simulink model "s_func_drone_vid2_fastest"
settings: Solver=FixedStepDiscrete  StartTime=0.0  StopTime=inf  FixedStep=0.05  RelTol=1e-3
libraries: etargetslib x12, dspnetwork x9, xpcseriallib x7, dspmtrx3 x4, visionsinks x1
settings Model: Creator=Ballistyx  LastModifiedBy=JLEE
settings DataIOCC: LimitDataPoints=on  SaveFormat=Array  SignalLoggingSaveFormat=ModelDataLogs  ReturnWorkspaceOutputs=off
settings OptimizationCC: ExpressionDepthLimit=2147483647  LifeSpan=inf  SimCompilerOptimization=Off
settings DebuggingCC: UnderspecifiedInitializationDetection=Classic  MergeDetectMultiDrivingBlocksExec=none  SolverPrmCheckMsg=warning  MultiTaskDSMMsg=warning  MultiTaskCondExecSysMsg=none  FcnCallInpInsideContextMsg=Enable All  FrameProcessingCompatibilityMsg=warning  StateNameClashWarn=warning  StrictBusMsg=None  SFUnexpectedBacktrackingDiag=warning  SFNoUnconditionalDefaultTransitionDiag=warning
settings HardwareCC: ProdBitPerPointer=32  ProdLargestAtomicFloat=None  ProdIntDivRoundTo=Undefined  ProdEndianess=Unspecified  ProdWordSize=32  ProdHWDeviceType=32-bit Generic
settings ModelReferenceCC: PropagateSignalLabelsOutOfModel=off
settings SFSimCC: SimUseLocalCustomCode=off
settings RTWCC: RTWUseLocalCustomCode=off  IncludeERTFirstTime=on  RTWCompilerOptimization=Off
settings CodeAppCC: CustomSymbolStrType=$N$R$M
settings GRTTargetCC: CodeReplacementLibrary=ANSI_C  GeneratePreprocessorConditionals=Disable all  CPPClassGenCompliant=off

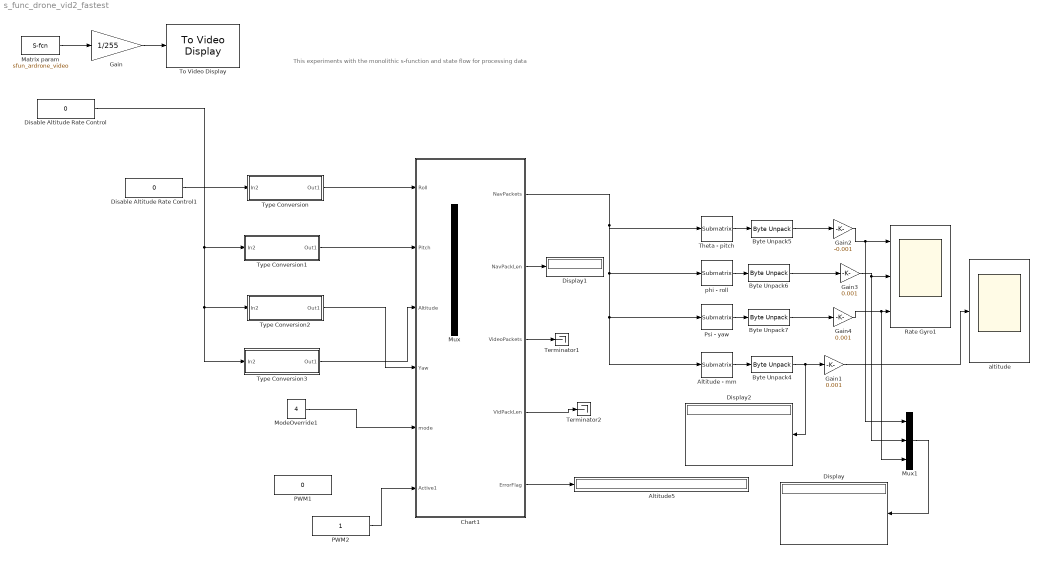
== system s_func_drone_vid2_fastest ==
  note: This experiments with the monolithic s-function and state flow for processing data
  Altitude - mm : dspmtrx3/Submatrix  RowSpan=Range of rows  RowStartMode=Index  RowStartIndex=41  RowEndMode=Index  RowEndIndex=44  ColSpan=All columns  ColStartMode=Index  ColStartIndex=4  ColEndMode=Index  ColEndIndex=4
  Altitude5 : Display
  Byte Unpack4 : etargetslib/Byte Unpack  dimensions={[1]}  datatypes={'uint32'}  byteAlign=1
  Byte Unpack5 : etargetslib/Byte Unpack  dimensions={[1]}  datatypes={'single'}  byteAlign=1
  Byte Unpack6 : etargetslib/Byte Unpack  dimensions={[1]}  datatypes={'single'}  byteAlign=1
  Byte Unpack7 : etargetslib/Byte Unpack  dimensions={[1]}  datatypes={'single'}  byteAlign=1
  Chart1 : Stateflow chart  TreatAsAtomicUnit=on
  Disable Altitude Rate Control : Constant  Value=0
  Disable Altitude Rate Control1 : Constant  Value=0
  Display : Display
  Display1 : Display
  Display2 : Display
  Gain : Gain  Gain=1/255
  Gain1 : Gain  Gain=0.001
  Gain2 : Gain  Gain=-0.001
  Gain3 : Gain  Gain=0.001
  Gain4 : Gain  Gain=0.001
  Matrix param : S-Function  FunctionName=sfun_ardrone_video  Parameters=Operand  EnableBusSupport=off  mask(Matrix add){Operand=4}
      mask prompts: Operand "Operand 1:"
      settings: AttributesFormatString=Param = %<Operand>
      mask Display: disp('Matrix\n Add ')
  ModeOverride1 : Constant  Value=4
  Mux : Mux
  Mux1 : Mux  Inputs=3
  PWM1 : Constant  Value=0
  PWM2 : Constant
  Psi - yaw : dspmtrx3/Submatrix  RowSpan=Range of rows  RowStartMode=Index  RowStartIndex=37  RowEndMode=Index  RowEndIndex=40  ColSpan=All columns  ColStartMode=Index  ColStartIndex=4  ColEndMode=Index  ColEndIndex=4
  Rate Gyro1 : Scope  NumInputPorts=3
      settings: YMin=0.295~2.935~32.9  YMax=0.365~3~34.4  SaveName=NavData_Simulink1
  Terminator1 : Terminator
  Terminator2 : Terminator
  Theta - pitch : dspmtrx3/Submatrix  RowSpan=Range of rows  RowStartMode=Index  RowStartIndex=29  RowEndMode=Index  RowEndIndex=32  ColSpan=All columns  ColStartMode=Index  ColStartIndex=4  ColEndMode=Index  ColEndIndex=4
  To Video Display : visionsinks/To Video Display  inputType=Obsolete  imagePorts=One multidimensional signal  OutputDevice=On-screen video monitor  fullScreen=off  videoWindowX=223  videoWindowY=316  saveWindowSize=off  videoWindowWidth=320  videoWindowHeight=240  dataOrg=Column-major  openAtMdlStart=on  isWindowOpen=on  inputColorFormat=RGB
  Type Conversion : Subsystem
  Type Conversion1 : Subsystem
  Type Conversion2 : Subsystem
  Type Conversion3 : Subsystem
  altitude : Scope
      settings: YMin=0.242  YMax=0.242  SaveName=NavData_Simulink
  phi - roll : dspmtrx3/Submatrix  RowSpan=Range of rows  RowStartMode=Index  RowStartIndex=33  RowEndMode=Index  RowEndIndex=36  ColSpan=All columns  ColStartMode=Index  ColStartIndex=4  ColEndMode=Index  ColEndIndex=4
  wires:
  Matrix param/1 -> Gain/1
  Gain/1 -> To Video Display/1
  Altitude - mm/1 -> Byte Unpack4/1
  Theta - pitch/1 -> Byte Unpack5/1
  phi - roll/1 -> Byte Unpack6/1
  Psi - yaw/1 -> Byte Unpack7/1
  Byte Unpack5/1 -> Gain2/1
  Byte Unpack6/1 -> Gain3/1
  Byte Unpack7/1 -> Gain4/1
  Byte Unpack4/1 -> Gain1/1, Display2/1
  Gain1/1 -> altitude/1
  Gain2/1 -> Rate Gyro1/1, Mux1/1
  Gain3/1 -> Rate Gyro1/2, Mux1/2
  Gain4/1 -> Rate Gyro1/3, Mux1/3
  PWM2/1 -> Chart1/6(Active1)
  Chart1/4(VidPackLen) -> Terminator2/1
  Chart1/5(ErrorFlag) -> Altitude5/1
  Type Conversion3/1(Out1) -> Chart1/3(Altitude)
  Type Conversion2/1(Out1) -> Chart1/4(Yaw)
  Type Conversion1/1(Out1) -> Chart1/2(Pitch)
  Type Conversion/1(Out1) -> Chart1/1(Roll)
  Disable Altitude Rate Control1/1 -> Type Conversion/1(In2)
  Disable Altitude Rate Control/1 -> Type Conversion1/1(In2), Type Conversion3/1(In2), Type Conversion2/1(In2)
  ? -> ?
  ModeOverride1/1 -> Chart1/5(mode)
  Chart1/2(NavPackLen) -> Display1/1
  Chart1/3(VideoPackets) -> Terminator1/1
  Chart1/1(NavPackets) -> Theta - pitch/1, phi - roll/1, Psi - yaw/1, Altitude - mm/1
  Mux1/1 -> Display/1

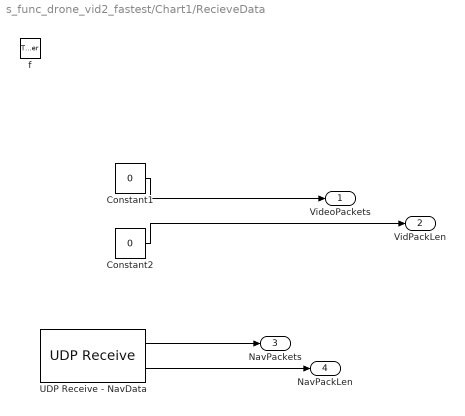
== system s_func_drone_vid2_fastest/Chart1/RecieveData ==
  f : TriggerPort  TriggerType=function-call
      settings: CopyFcn=Stateflow.SLINSF.SimulinkMan.removeBlockPreDeleteFcn  PreDeleteFcn=Stateflow.SLINSF.SimulinkMan.unsafePredeleteFcn
  Constant1 : Constant  Value=0
  Constant2 : Constant  Value=0
  UDP Receive - NavData : dspnetwork/UDP Receive  Priority=11  localURL='0.0.0.0'  localPort=5554  remoteURL='192.168.1.1'  remotePort=-1  recvBufferSize=500  dims=500  signalDatatype=uint8  isVarSize=off  showBlockingTime=off  blockingTime=0  sampletime=-1
  VideoPackets : Outport
  VidPackLen : Outport  Port=2
  NavPackets : Outport  Port=3
  NavPackLen : Outport  Port=4
  wires:
  Constant1/1 -> VideoPackets/1
  Constant2/1 -> VidPackLen/1
  UDP Receive - NavData/1 -> NavPackets/1
  UDP Receive - NavData/2 -> NavPackLen/1

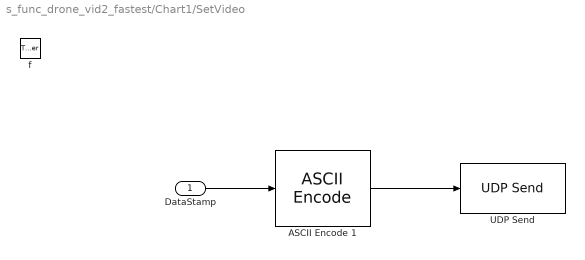
== system s_func_drone_vid2_fastest/Chart1/SetVideo ==
  DataStamp : Inport
  f : TriggerPort  TriggerType=function-call
      settings: CopyFcn=Stateflow.SLINSF.SimulinkMan.removeBlockPreDeleteFcn  PreDeleteFcn=Stateflow.SLINSF.SimulinkMan.unsafePredeleteFcn
  ASCII Encode 1 : xpcseriallib/ASCII Encode   format="AT*CONFIG=%d,\\\"video:video_channel\\\",\\\"0\\\"\\r"  nvars=1  maxlength=44  vartypes={ 'uint32' }
  UDP Send : dspnetwork/UDP Send  remoteURL='192.168.1.1'  remotePort=5556  localURL='0.0.0.0'  localPortSource=Specify via dialog  localPort=5556  sampletime=-1  separateLengthPort=0
  wires:
  DataStamp/1 -> ASCII Encode 1/1
  ASCII Encode 1/1 -> UDP Send/1

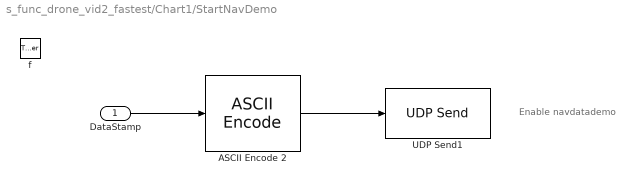
== system s_func_drone_vid2_fastest/Chart1/StartNavDemo ==
  note: Enable navdatademo
  DataStamp : Inport
  f : TriggerPort  TriggerType=function-call
      settings: CopyFcn=Stateflow.SLINSF.SimulinkMan.removeBlockPreDeleteFcn  PreDeleteFcn=Stateflow.SLINSF.SimulinkMan.unsafePredeleteFcn
  ASCII Encode 2 : xpcseriallib/ASCII Encode   format="AT*CONFIG=%d,\\\"general:navdata_demo\\\",\\\"TRUE\\\"\\r"  nvars=1  maxlength=43  vartypes={ 'uint32' }
  UDP Send1 : dspnetwork/UDP Send  remoteURL='192.168.1.1'  remotePort=5556  localURL='0.0.0.0'  localPortSource=Specify via dialog  localPort=5556  sampletime=-1  separateLengthPort=0
  wires:
  DataStamp/1 -> ASCII Encode 2/1
  ASCII Encode 2/1 -> UDP Send1/1

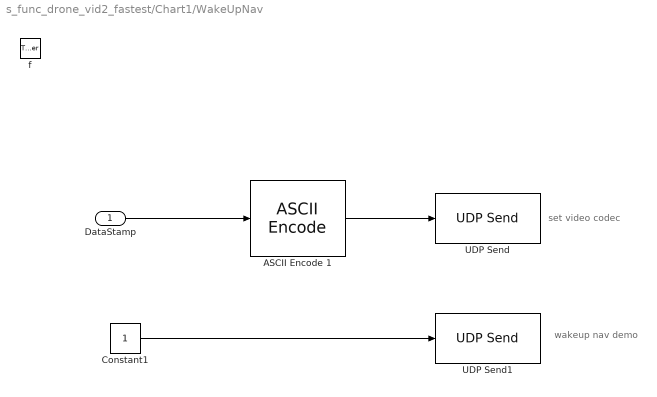
== system s_func_drone_vid2_fastest/Chart1/WakeUpNav ==
  note: set video codec
  note: wakeup nav demo
  DataStamp : Inport
  f : TriggerPort  TriggerType=function-call
      settings: CopyFcn=Stateflow.SLINSF.SimulinkMan.removeBlockPreDeleteFcn  PreDeleteFcn=Stateflow.SLINSF.SimulinkMan.unsafePredeleteFcn
  ASCII Encode 1 : xpcseriallib/ASCII Encode   format="AT*CONFIG=%d,\\\"video:video_codec\\\",\\\"32\\\"\\r"  nvars=1  maxlength=44  vartypes={ 'uint32' }
  Constant1 : Constant  OutDataTypeStr=uint8  SampleTime=-1
  UDP Send : dspnetwork/UDP Send  remoteURL='192.168.1.1'  remotePort=5556  localURL='0.0.0.0'  localPortSource=Specify via dialog  localPort=5556  sampletime=-1  separateLengthPort=0
  UDP Send1 : dspnetwork/UDP Send  remoteURL='192.168.1.1'  remotePort=5554  localURL='0.0.0.0'  localPortSource=Specify via dialog  localPort=5554  sampletime=-1  separateLengthPort=0
  wires:
  DataStamp/1 -> ASCII Encode 1/1
  Constant1/1 -> UDP Send1/1
  ASCII Encode 1/1 -> UDP Send/1

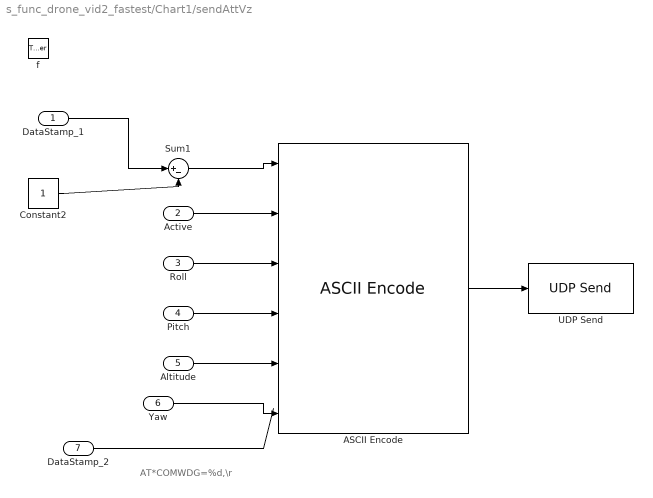
== system s_func_drone_vid2_fastest/Chart1/sendAttVz ==
  note: AT*COMWDG=%d,\r
  DataStamp_1 : Inport
  Active : Inport  Port=2
  Roll : Inport  Port=3
  Pitch : Inport  Port=4
  Altitude : Inport  Port=5
  Yaw : Inport  Port=6
  DataStamp_2 : Inport  Port=7
  f : TriggerPort  TriggerType=function-call
      settings: CopyFcn=Stateflow.SLINSF.SimulinkMan.removeBlockPreDeleteFcn  PreDeleteFcn=Stateflow.SLINSF.SimulinkMan.unsafePredeleteFcn
  "ASCII Encode " : xpcseriallib/ASCII Encode   format=AT*PCMD=%d,%d,%d,%d,%d,%d\r  nvars=6  maxlength=128  vartypes={ 'double' }
  Constant2 : Constant
  Sum1 : Sum  Inputs=|+-
  UDP Send : dspnetwork/UDP Send  remoteURL='192.168.1.1'  remotePort=5556  localURL='0.0.0.0'  localPortSource=Specify via dialog  localPort=5556  sampletime=-1  separateLengthPort=0
  wires:
  Active/1 -> "ASCII Encode "/2
  Roll/1 -> "ASCII Encode "/3
  Pitch/1 -> "ASCII Encode "/4
  Altitude/1 -> "ASCII Encode "/5
  Yaw/1 -> "ASCII Encode "/6
  DataStamp_2/1 -> ?
  DataStamp_1/1 -> Sum1/1
  Sum1/1 -> "ASCII Encode "/1
  Constant2/1 -> Sum1/2
  "ASCII Encode "/1 -> UDP Send/1

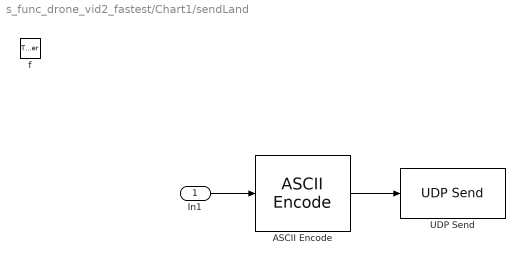
== system s_func_drone_vid2_fastest/Chart1/sendLand ==
  In1 : Inport
  f : TriggerPort  TriggerType=function-call
      settings: CopyFcn=Stateflow.SLINSF.SimulinkMan.removeBlockPreDeleteFcn  PreDeleteFcn=Stateflow.SLINSF.SimulinkMan.unsafePredeleteFcn
  "ASCII Encode " : xpcseriallib/ASCII Encode   format=AT*REF=%d,290717696\r  nvars=1  maxlength=128  vartypes={ 'double' }
  UDP Send : dspnetwork/UDP Send  remoteURL='192.168.1.1'  remotePort=5556  localURL='0.0.0.0'  localPortSource=Specify via dialog  localPort=5556  sampletime=-1  separateLengthPort=0
  wires:
  "ASCII Encode "/1 -> UDP Send/1
  In1/1 -> "ASCII Encode "/1

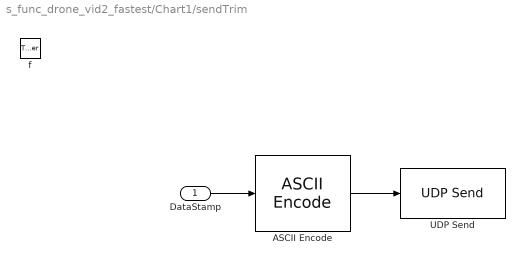
== system s_func_drone_vid2_fastest/Chart1/sendTrim ==
  DataStamp : Inport
  f : TriggerPort  TriggerType=function-call
      settings: CopyFcn=Stateflow.SLINSF.SimulinkMan.removeBlockPreDeleteFcn  PreDeleteFcn=Stateflow.SLINSF.SimulinkMan.unsafePredeleteFcn
  "ASCII Encode " : xpcseriallib/ASCII Encode   format=AT*FTRIM=%d,\r  nvars=1  maxlength=128  vartypes={ 'double' }
  UDP Send : dspnetwork/UDP Send  remoteURL='192.168.1.1'  remotePort=5556  localURL='0.0.0.0'  localPortSource=Specify via dialog  localPort=5556  sampletime=-1  separateLengthPort=0
  wires:
  "ASCII Encode "/1 -> UDP Send/1
  DataStamp/1 -> "ASCII Encode "/1

== system s_func_drone_vid2_fastest/Chart1/startHover ==
  note: disable hover for now
  DataStamp : Inport
  f : TriggerPort  TriggerType=function-call
      settings: CopyFcn=Stateflow.SLINSF.SimulinkMan.removeBlockPreDeleteFcn  PreDeleteFcn=Stateflow.SLINSF.SimulinkMan.unsafePredeleteFcn
  "ASCII Encode " : xpcseriallib/ASCII Encode   format=AT*REF=%d,290718208\r  nvars=1  maxlength=128  vartypes={ 'double' }
  UDP Send : dspnetwork/UDP Send  remoteURL='192.168.1.1'  remotePort=5556  localURL='0.0.0.0'  localPortSource=Specify via dialog  localPort=5556  sampletime=-1  separateLengthPort=0
  wires:
  DataStamp/1 -> "ASCII Encode "/1

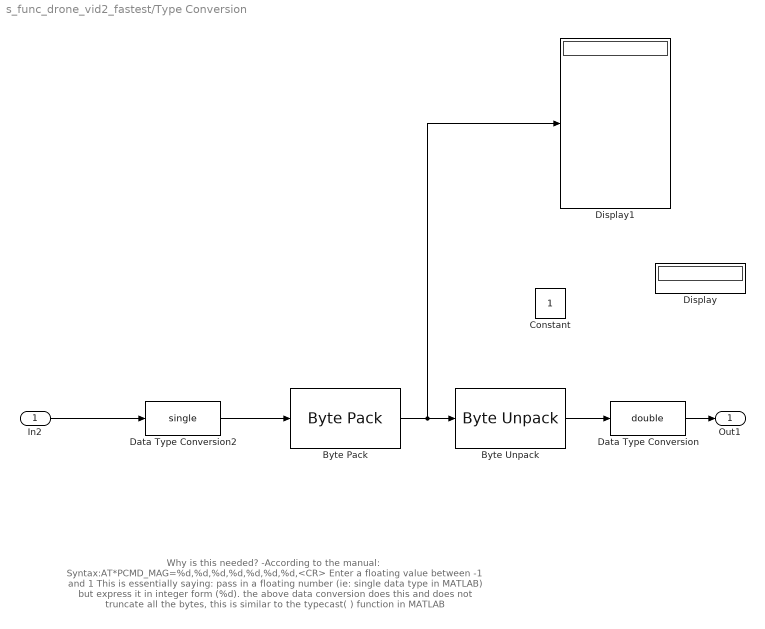
== system s_func_drone_vid2_fastest/Type Conversion ==
  note: Why is this needed?
      | -According to the manual:
      |
      | Syntax:AT*PCMD_MAG=%d,%d,%d,%d,%d,%d,%d,<CR>
      | Enter a floating value between -1 and 1
      |
      | This is essentially saying: pass in a floating number (ie: single data type in MATLAB) but express it in integer form (%d).
      | the above data conversion does this and does not truncate all the bytes, this is similar to the typecast( ) function in MATLAB
  In2 : Inport
  Byte Pack : etargetslib/Byte Pack  datatypes={'single'}  byteAlign=1
  Byte Unpack : etargetslib/Byte Unpack  dimensions={[1]}  datatypes={'int32'}  byteAlign=1
  Constant : Constant
  Data Type Conversion : DataTypeConversion  OutDataTypeStr=double
  Data Type Conversion2 : DataTypeConversion  OutDataTypeStr=single
  Display : Display
  Display1 : Display
  Out1 : Outport
  wires:
  In2/1 -> Data Type Conversion2/1
  Data Type Conversion2/1 -> Byte Pack/1
  Data Type Conversion/1 -> Out1/1
  Byte Pack/1 -> Byte Unpack/1, Display1/1
  Byte Unpack/1 -> Data Type Conversion/1
  ? -> Display/1

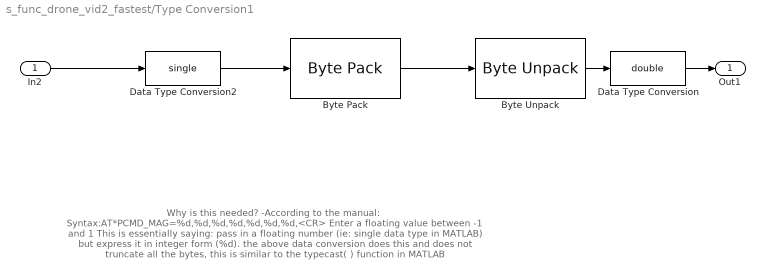
== system s_func_drone_vid2_fastest/Type Conversion1 ==
  note: Why is this needed?
      | -According to the manual:
      |
      | Syntax:AT*PCMD_MAG=%d,%d,%d,%d,%d,%d,%d,<CR>
      | Enter a floating value between -1 and 1
      |
      | This is essentially saying: pass in a floating number (ie: single data type in MATLAB) but express it in integer form (%d).
      | the above data conversion does this and does not truncate all the bytes, this is similar to the typecast( ) function in MATLAB
  In2 : Inport
  Byte Pack : etargetslib/Byte Pack  datatypes={'single'}  byteAlign=1
  Byte Unpack : etargetslib/Byte Unpack  dimensions={[1]}  datatypes={'int32'}  byteAlign=1
  Data Type Conversion : DataTypeConversion  OutDataTypeStr=double
  Data Type Conversion2 : DataTypeConversion  OutDataTypeStr=single
  Out1 : Outport
  wires:
  Byte Pack/1 -> Byte Unpack/1
  Byte Unpack/1 -> Data Type Conversion/1
  In2/1 -> Data Type Conversion2/1
  Data Type Conversion2/1 -> Byte Pack/1
  Data Type Conversion/1 -> Out1/1

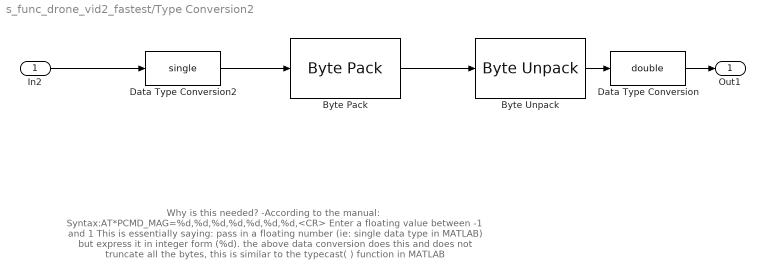
== system s_func_drone_vid2_fastest/Type Conversion2 ==
  note: Why is this needed?
      | -According to the manual:
      |
      | Syntax:AT*PCMD_MAG=%d,%d,%d,%d,%d,%d,%d,<CR>
      | Enter a floating value between -1 and 1
      |
      | This is essentially saying: pass in a floating number (ie: single data type in MATLAB) but express it in integer form (%d).
      | the above data conversion does this and does not truncate all the bytes, this is similar to the typecast( ) function in MATLAB
  In2 : Inport
  Byte Pack : etargetslib/Byte Pack  datatypes={'single'}  byteAlign=1
  Byte Unpack : etargetslib/Byte Unpack  dimensions={[1]}  datatypes={'int32'}  byteAlign=1
  Data Type Conversion : DataTypeConversion  OutDataTypeStr=double
  Data Type Conversion2 : DataTypeConversion  OutDataTypeStr=single
  Out1 : Outport
  wires:
  Byte Pack/1 -> Byte Unpack/1
  Byte Unpack/1 -> Data Type Conversion/1
  In2/1 -> Data Type Conversion2/1
  Data Type Conversion2/1 -> Byte Pack/1
  Data Type Conversion/1 -> Out1/1

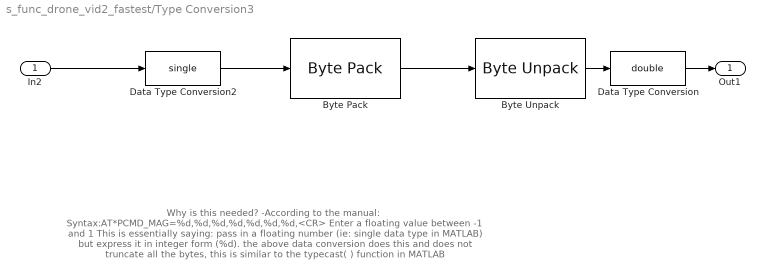
== system s_func_drone_vid2_fastest/Type Conversion3 ==
  note: Why is this needed?
      | -According to the manual:
      |
      | Syntax:AT*PCMD_MAG=%d,%d,%d,%d,%d,%d,%d,<CR>
      | Enter a floating value between -1 and 1
      |
      | This is essentially saying: pass in a floating number (ie: single data type in MATLAB) but express it in integer form (%d).
      | the above data conversion does this and does not truncate all the bytes, this is similar to the typecast( ) function in MATLAB
  In2 : Inport
  Byte Pack : etargetslib/Byte Pack  datatypes={'single'}  byteAlign=1
  Byte Unpack : etargetslib/Byte Unpack  dimensions={[1]}  datatypes={'int32'}  byteAlign=1
  Data Type Conversion : DataTypeConversion  OutDataTypeStr=double
  Data Type Conversion2 : DataTypeConversion  OutDataTypeStr=single
  Out1 : Outport
  wires:
  Byte Pack/1 -> Byte Unpack/1
  Byte Unpack/1 -> Data Type Conversion/1
  In2/1 -> Data Type Conversion2/1
  Data Type Conversion2/1 -> Byte Pack/1
  Data Type Conversion/1 -> Out1/1

== stateflow chart s_func_drone_vid2_fastest/Chart1 ==
  state ExecuteTrimCmd_State
    entry:ErrorFlag = 0;
    during: sendTrim(i)
  state ModeSelector
  state sendTrim(DataStamp) [function]
  state WakeUpNavVideo_State
    entry:ErrorFlag = 0;
    during: WakeUpNav(i)
  state WakeUpNav(DataStamp) [function]
  state StartNavDemo_State
    entry:ErrorFlag = 0;
    during: StartNavDemo(i)
  state StartNavDemo(DataStamp) [function]
  state SetVideoChannel_State
    entry:ErrorFlag = 0;
    during: SetVideo(i)
  state SetVideo(DataStamp) [function]
  state BeginHover_State
    entry:ErrorFlag = 0;
    during: startHover(i)
  state startHover(DataStamp) [function]
  state Control_State
    entry:ErrorFlag = 0;
    entry: sendAttVz(i,Active1,Roll,Pitch,Altitude,Yaw,i)
  state RunMotor6
    entry:ErrorFlag = 0;
    during: sendLand(i)
  state sendAttVz(DataStamp_1,Active,Roll,Pitch,Altitude,Yaw,DataStamp_2) [function]
  state sendLand(In1) [function]
  state RecieveData_State
    entry:     [VideoPackets,VidPackLen,NavPackets,NavPackLen]  = RecieveData()
  state [VideoPackets,VidPackLen,NavPackets,NavPackLen] = RecieveData [function]
  (default) -> (junction 7)
  (junction 7) -> ModeSelector : {i = 1}
  ExecuteTrimCmd_State -> ModeSelector [order 1] : [mode~=4]
  ModeSelector -> ExecuteTrimCmd_State : [mode == 4]
      | {i=i+1;}
  ExecuteTrimCmd_State -> WakeUpNavVideo_State [order 2] : after(3,sec)
      | {i=i+1;}
  RunMotor6 -> ModeSelector : after(1,sec)
  WakeUpNavVideo_State -> StartNavDemo_State : after(1,sec)
      | {i = i +1;}
  StartNavDemo_State -> SetVideoChannel_State : after(0.1,sec)
      | {i=i+1;}
  SetVideoChannel_State -> BeginHover_State : after(0.1,sec)
      | {i =i +1;}
  BeginHover_State -> Control_State : after(1,sec)
      | {i=i+2;}
  Control_State -> RunMotor6 [order 1] : [mode~=4]
      | {i=i+1;}
  Control_State -> RecieveData_State [order 2] : after(0.05,sec)
      | {i=i+1;}
  RecieveData_State -> Control_State : after(0.05,sec)
      | {i=i+2;}
  data: DataStamp function_input; DataStamp function_input; DataStamp function_input; DataStamp function_input; DataStamp function_input; DataStamp_1 function_input; Active function_input; Roll function_input; Pitch function_input; Altitude function_input; Yaw function_input; DataStamp_2 function_input; In1 function_input; VideoPackets function_output; VidPackLen function_output; NavPackets function_output; NavPackLen function_output; Roll input double; Pitch input double; Altitude input double; Yaw input double; mode input; i local double; NavPackets output uint8 size=[500,1]; NavPackLen output double; VideoPackets output uint8 size=[40000,1]; VidPackLen output double; ErrorFlag output double; Active1 input double
